simulink model "MainEngine"  (R2024b)
settings: Solver=ode4  StartTime=0.0  StopTime=600  FixedStep=0.01  RelTol=1e-3
undefined symbols (not defined in the file): g0, LLM
settings Model: DVExtractedSubsystem=Main Engine  DVDesignModelName=simulation  Creator=simon  LastModifiedBy=simon
settings DebuggingCC: FrameProcessingCompatibilityMsg=none
settings RTWCC: TLCOptions=-aAlwaysIncludeCustomSrc=1

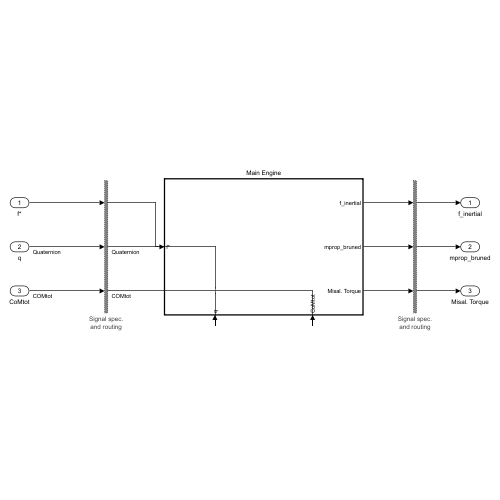
[thumbnail: Simulink's stored preview of the top-level diagram]
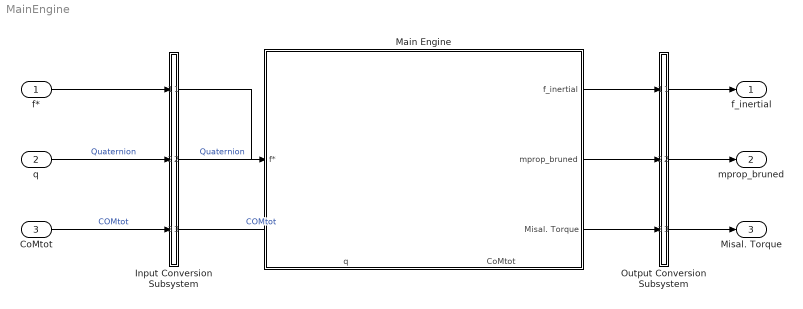
== system MainEngine ==
  f* : Inport  OutDataTypeStr=double  PortDimensions=[3, 1]  Interpolate=off
  q : Inport  Port=2  OutDataTypeStr=double  PortDimensions=[4, 1]  Interpolate=off
  CoMtot : Inport  Port=3  OutDataTypeStr=double  PortDimensions=[3]  Interpolate=off
  Input Conversion Subsystem : Subsystem  Tag=__SLT_ICS__  Description=|
      | Signal spec.
      | and routing
      settings: AttributesFormatString=%<Description>
  Main Engine : Subsystem  TreatAsAtomicUnit=on
      settings: PortSchema="{\"entries\":[{\"content\":{\"sides\":[{\"content\":{\"connectorIds\":[\"In1\"]},\"type\":\"ConnectorPlacement.EquallySpacedRectSide\",\"uuid\":\"1cd70ed7-fffe-4052-be12-d08ec438809a\"},{\"content\":{\"connectorIds\":[\"Out1\",\"Out2\",\"Out3\"],\"side\":\"RIGHT\"},\"type\":\"ConnectorPlacement.EquallySpacedRectSide\",\"uuid\":\"572c642b-d704-4725-a3d6-bfccbd3ff261\"},{\"content\":{\"side\":\"TOP\"},\"type\":\"ConnectorPlacement.EquallySpacedRectSide\",\"uuid\":\"96cefc9d-2b60-4f61-9fb0-422319e028d1\"},{\"content\":{\"connectorIds\":[\"In2\",\"In3\"],\"side\":\"BOTTOM\"},\"type\":\"ConnectorPlacement.EquallySpacedRectSide\",\"uuid\":\"b823879b-ffc4-494b-bbd8-898eb74a4cd3\"}]},\"type\":\"ConnectorPlacement.EquallySpacedConnector\",\"uuid\":\"14908dc7-5499-48fd-923a-6110af65b868\"}],\"packageUris\":[\"http://schema.mathworks.com/mf0/Connector/R2020b\"],\"version\":\"1.0\"}"
  Output Conversion Subsystem : Subsystem  Tag=__SLT_OCS__  Description=|
      | Signal spec.
      | and routing
      settings: AttributesFormatString=%<Description>
  f_inertial : Outport
  mprop_bruned : Outport  Port=2
  Misal. Torque : Outport  Port=3
  wires:
  f*/1 -> Input Conversion Subsystem/1(Inport_1)
  q/1 -> Input Conversion Subsystem/2(Inport_2)  "Quaternion"
  CoMtot/1 -> Input Conversion Subsystem/3(Inport_3)  "COMtot"
  Output Conversion Subsystem/1(Outport_1) -> f_inertial/1
  Output Conversion Subsystem/2(Outport_2) -> mprop_bruned/1
  Output Conversion Subsystem/3(Outport_3) -> Misal. Torque/1
  Input Conversion Subsystem/1(Outport_1) -> Main Engine/1(f*)
  Input Conversion Subsystem/2(Outport_2) -> Main Engine/2(q)  "Quaternion"
  Input Conversion Subsystem/3(Outport_3) -> Main Engine/3(CoMtot)  "COMtot"
  Main Engine/1(f_inertial) -> Output Conversion Subsystem/1(Inport_1)
  Main Engine/2(mprop_bruned) -> Output Conversion Subsystem/2(Inport_2)
  Main Engine/3(Misal. Torque) -> Output Conversion Subsystem/3(Inport_3)

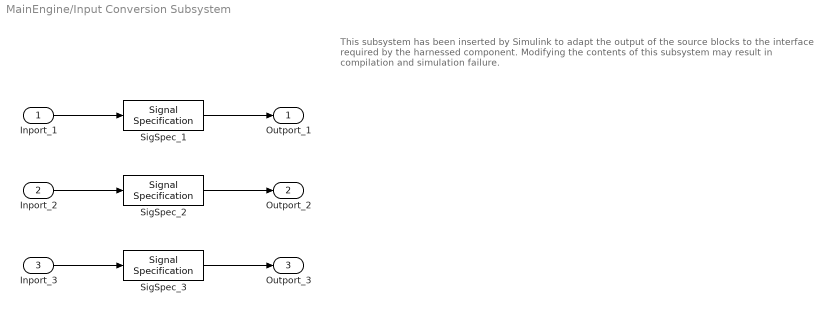
== system MainEngine/Input Conversion Subsystem ==
  note: This subsystem has been inserted by Simulink to adapt the output of the source blocks to the interface required by the harnessed component.
      |  Modifying the contents of this subsystem may result in compilation and simulation failure.
  Inport_1 : Inport
  Inport_2 : Inport  Port=2
  Inport_3 : Inport  Port=3
  SigSpec_1 : SignalSpecification  OutDataTypeStr=double  Dimensions=[3, 1]
  SigSpec_2 : SignalSpecification  OutDataTypeStr=double  Dimensions=[4, 1]
  SigSpec_3 : SignalSpecification  OutDataTypeStr=double  Dimensions=[3]
  Outport_1 : Outport
  Outport_2 : Outport  Port=2
  Outport_3 : Outport  Port=3
  wires:
  SigSpec_1/1 -> Outport_1/1
  Inport_1/1 -> SigSpec_1/1
  SigSpec_2/1 -> Outport_2/1
  Inport_2/1 -> SigSpec_2/1
  SigSpec_3/1 -> Outport_3/1
  Inport_3/1 -> SigSpec_3/1

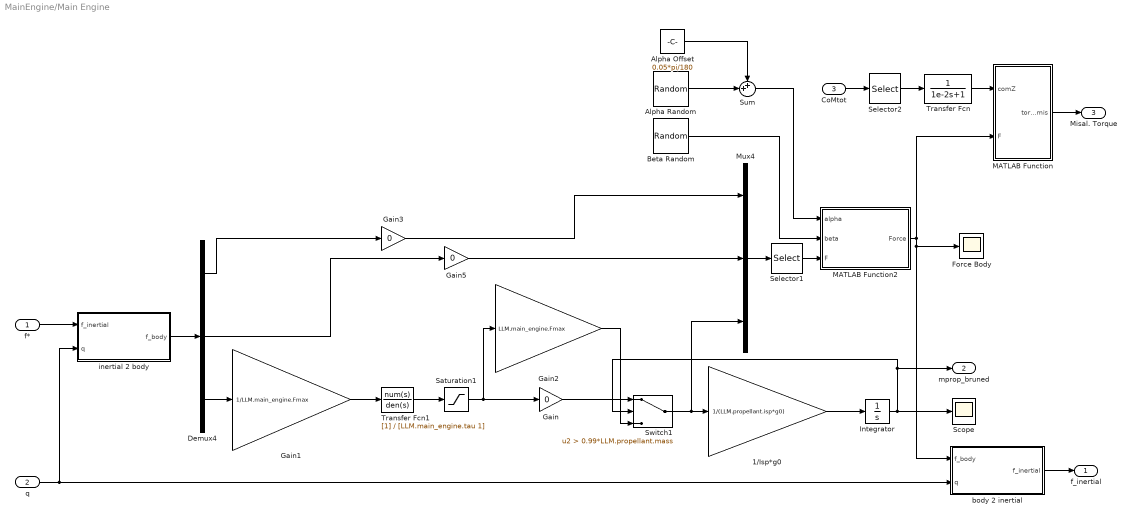
== system MainEngine/Main Engine ==
  f* : Inport
  q : Inport  Port=2
  CoMtot : Inport  Port=3
  1/Isp*g0 : Gain  Gain=1/(LLM.propellant.isp*g0)
  Alpha Offset : Constant  Value=0.05*pi/180
  Alpha Random : UniformRandomNumber  Minimum=-LLM.main_engine.misallignment_alpha*pi/180  Maximum=LLM.main_engine.misallignment_alpha*pi/180  SampleTime=0.1
  Beta Random : UniformRandomNumber  Minimum=-LLM.main_engine.misallignment_beta*pi/180  Maximum=LLM.main_engine.misallignment_beta*pi/180  Seed=1  SampleTime=0.1
  Demux4 : Demux  Outputs=3
  Force Body : Scope
  Gain : Gain  Gain=0
  Gain1 : Gain  Gain=1/LLM.main_engine.Fmax
  Gain2 : Gain  Gain=LLM.main_engine.Fmax
  Gain3 : Gain  Gain=0
  Gain5 : Gain  Gain=0
  Integrator : Integrator  LimitOutput=on  UpperSaturationLimit=LLM.propellant.mass  LowerSaturationLimit=0
  MATLAB Function : MATLAB Function  TreatAsAtomicUnit=on
  MATLAB Function2 : MATLAB Function  TreatAsAtomicUnit=on
  Mux4 : Mux  Inputs=3
  Saturation1 : Saturate  UpperLimit=1  LowerLimit=-1
  Scope : Scope
  Selector1 : Selector  InputPortWidth=3  IndexOptions=Index vector (dialog)  Indices=[3]  OutputSizes=1
  Selector2 : Selector  InputPortWidth=3  IndexOptions=Index vector (dialog)  Indices=[3]  OutputSizes=1
  Sum : Sum  Inputs=++|
  Switch1 : Switch  Criteria=u2 > Threshold  Threshold=0.99*LLM.propellant.mass  SaturateOnIntegerOverflow=off  InputSameDT=off
  Transfer Fcn : TransferFcn  Denominator=[1e-2 1]
  Transfer Fcn1 : TransferFcn  Denominator=[LLM.main_engine.tau 1]
  body 2 inertial : MATLAB Function  TreatAsAtomicUnit=on
  inertial 2 body : MATLAB Function  TreatAsAtomicUnit=on
  f_inertial : Outport
  mprop_bruned : Outport  Port=2
  Misal. Torque : Outport  Port=3
  wires:
  Alpha Offset/1 -> Sum/1
  Sum/1 -> MATLAB Function2/1(alpha)
  Alpha Random/1 -> Sum/2
  Beta Random/1 -> MATLAB Function2/2(beta)
  Selector2/1 -> Transfer Fcn/1
  MATLAB Function/1(torque_mis) -> Misal. Torque/1
  MATLAB Function2/1(Force) -> Force Body/1, body 2 inertial/1(f_body), MATLAB Function/2(F)
  Transfer Fcn/1 -> MATLAB Function/1(comZ)
  CoMtot/1 -> Selector2/1
  Selector1/1 -> MATLAB Function2/3(F)
  body 2 inertial/1(f_inertial) -> f_inertial/1
  1/Isp*g0/1 -> Integrator/1
  Switch1/1 -> 1/Isp*g0/1, Mux4/3
  Gain/1 -> Switch1/1
  Saturation1/1 -> Gain/1, Gain2/1
  Mux4/1 -> Selector1/1
  Gain5/1 -> Mux4/2
  Integrator/1 -> Scope/1, mprop_bruned/1, Switch1/2
  Transfer Fcn1/1 -> Saturation1/1
  Gain3/1 -> Mux4/1
  Gain1/1 -> Transfer Fcn1/1
  Demux4/1 -> Gain3/1
  inertial 2 body/1(f_body) -> Demux4/1
  Demux4/3 -> Gain1/1
  Demux4/2 -> Gain5/1
  q/1 -> inertial 2 body/2(q), body 2 inertial/2(q)
  Gain2/1 -> Switch1/3
  f*/1 -> inertial 2 body/1(f_inertial)

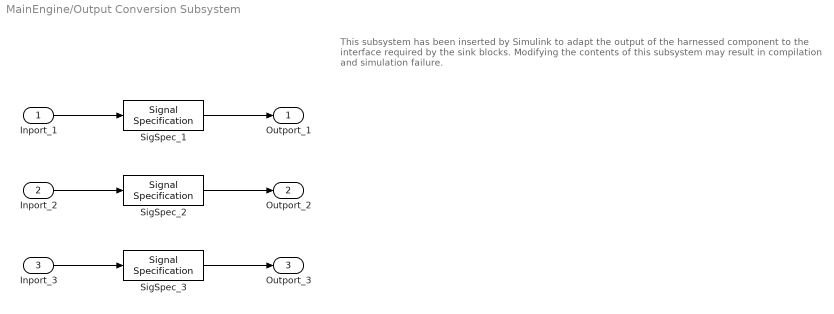
== system MainEngine/Output Conversion Subsystem ==
  note: This subsystem has been inserted by Simulink to adapt the output of the harnessed component to the interface required by the sink blocks.
      |  Modifying the contents of this subsystem may result in compilation and simulation failure.
  Inport_1 : Inport
  Inport_2 : Inport  Port=2
  Inport_3 : Inport  Port=3
  SigSpec_1 : SignalSpecification  OutDataTypeStr=double  Dimensions=[3, 1]
  SigSpec_2 : SignalSpecification  OutDataTypeStr=double  Dimensions=[1]
  SigSpec_3 : SignalSpecification  OutDataTypeStr=double  Dimensions=[3, 1]
  Outport_1 : Outport
  Outport_2 : Outport  Port=2
  Outport_3 : Outport  Port=3
  wires:
  Inport_1/1 -> SigSpec_1/1
  SigSpec_1/1 -> Outport_1/1
  Inport_2/1 -> SigSpec_2/1
  SigSpec_2/1 -> Outport_2/1
  Inport_3/1 -> SigSpec_3/1
  SigSpec_3/1 -> Outport_3/1

== matlab function MainEngine/Main Engine/MATLAB Function2 ==
  data: alpha input; beta input; F input; Force output
function Force = ForceRotate(alpha, beta,F)
%#codegen
% ForceRotate
% Ruota la forza iniziale [0;0;F] usando angoli polari:
%   alpha = angolo tra il raggio e l'asse Z
%   beta  = azimut nel piano XY misurato da +X verso +Y
%
% INPUTS:
%   F          - modulo della forza (scalar o array)
%   alpha, beta- angoli (stesse dimensioni di F o scalari)
%   useDegrees - (opzionale) true se alpha/beta sono in gradi
% OUTPUTS:
%   Fx, Fy, Fz - componenti ruotate
%
% Formula:
%   Fx = F*sin(alpha)*cos(beta)
%   Fy = F*sin(alpha)*sin(beta)
%   Fz = F*cos(alpha)

sa = sin(alpha);   ca = cos(alpha);
sb = sin(beta);    cb = cos(beta);

Fx = F .* sa .* cb;
Fy = F .* sa .* sb;
Fz = F .* ca;

Force = [Fx;Fy;Fz];
end

== matlab function MainEngine/Main Engine/body 2 inertial ==
  data: f_body input; q input; f_inertial output
function f_inertial = fcn(f_body,q)

% Using quaternions
q0 = q(1);
q1 = q(2);
q2 = q(3);
q3 = q(4);
R = [q0^2+q1^2-q2^2-q3^2 2*(q1*q2-q0*q3) 2*(q1*q3+q0*q2);
     2*(q1*q2+q0*q3) q0^2-q1^2+q2^2-q3^2 2*(q2*q3-q0*q1);
     2*(q1*q3-q0*q2) 2*(q2*q3+q0*q1) q0^2-q1^2-q2^2+q3^2];


% Using euler angles (ZYX)
% eul(1) rotation around x
% eul(2) rotation around y'
% eul(3) rotation around z''
% Rx = @(thx) [1 0 0; 0 cos(thx) -sin(thx); 0 sin(thx) cos(thx)];
% Ry = @(thy) [cos(thy) 0 sin(thy); 0 1 0; -sin(thy) 0 cos(thy)];
% Rz = @(thz) [cos(thz) -sin(thz) 0; sin(thz) cos(thz) 0; 0 0 1];
% R = Rz(eul(3))*Ry(eul(2))*Rx(eul(1));
f_inertial = R'*f_body;

== matlab function MainEngine/Main Engine/inertial 2 body ==
  data: f_inertial input; q input; f_body output
function f_body = fcn(f_inertial,q)

% Using quaternions
q0 = q(1);
q1 = q(2);
q2 = q(3);
q3 = q(4);
R = [q0^2+q1^2-q2^2-q3^2 2*(q1*q2-q0*q3) 2*(q1*q3+q0*q2);
     2*(q1*q2+q0*q3) q0^2-q1^2+q2^2-q3^2 2*(q2*q3-q0*q1);
     2*(q1*q3-q0*q2) 2*(q2*q3+q0*q1) q0^2-q1^2-q2^2+q3^2];


% Using euler angles (ZYX)
% eul(1) rotation around x
% eul(2) rotation around y'
% eul(3) rotation around z''
% Rx = @(thx) [1 0 0; 0 cos(thx) -sin(thx); 0 sin(thx) cos(thx)];
% Ry = @(thy) [cos(thy) 0 sin(thy); 0 1 0; -sin(thy) 0 cos(thy)];
% Rz = @(thz) [cos(thz) -sin(thz) 0; sin(thz) cos(thz) 0; 0 0 1];
% R = Rz(eul(3))*Ry(eul(2))*Rx(eul(1));
f_body = R*f_inertial;

== matlab function MainEngine/Main Engine/MATLAB Function ==
  data: comZ input; torque_mis output; F input
function torque_mis = fcn(comZ, F)

torque_mis = [F(1)*comZ; F(2)*comZ; 0];
